simulink model "CylinderSim"  (R2015a)
settings: Solver=ode45  StartTime=0.0  StopTime=2.5  RelTol=1e-3
settings Model: CovSFcnEnable=off  Creator=jportella  LastModifiedBy=user
settings DebuggingCC: SolverPrmCheckMsg=warning

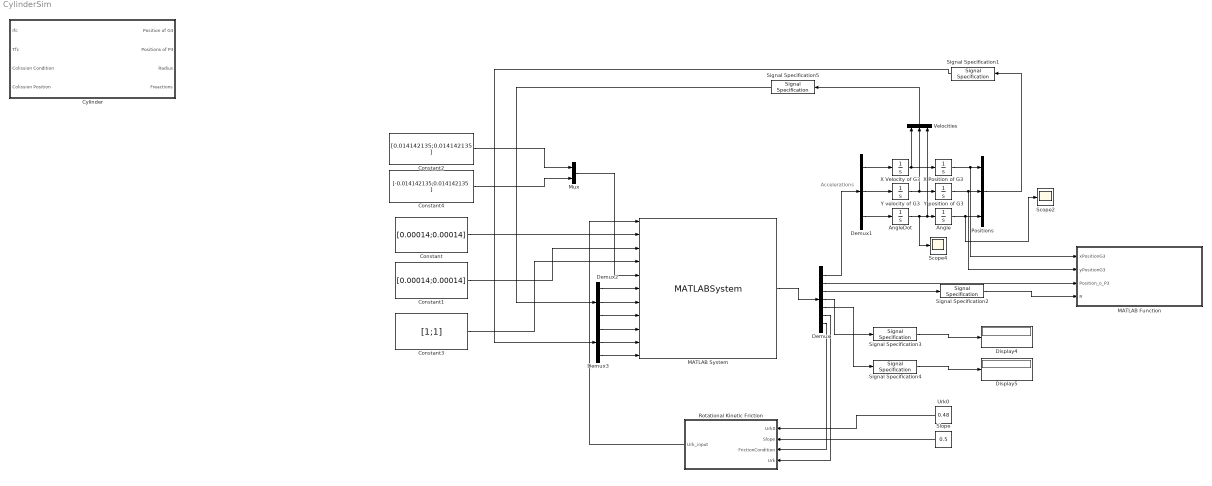
== system CylinderSim ==
  note: Accelerations
  Angle : Integrator
  AngleDot : Integrator
  Constant : Constant  Value=[0.00014;0.00014]
  Constant1 : Constant  Value=[0.00014;0.00014]
  Constant2 : Constant  Value=[0.014142135;0.014142135 ]
  Constant3 : Constant  Value=[1;1]
  Constant4 : Constant  Value=[-0.014142135;0.014142135 ]
  Cylinder : Subsystem
  Demux : Demux  Outputs=7
  Demux1 : Demux  Outputs=3
  Demux2 : Demux  Outputs=3
  Demux3 : Demux  Outputs=3
  Display4 : Display
  Display5 : Display
  MATLAB Function : MATLAB Function  TreatAsAtomicUnit=on
  MATLAB System : MATLABSystem  System=Cylinder  R=0.02  M=0.003  g=9.81  Us=0.5  Uk=0.48  Urs=0.5  Urk=0.48  Ucs=0.5  Uck=0.4  Iz=6.0000000000000008e-07  F_s_x=0.014715  F_s_y=0.014715  F_k_x=0.0141264  F_k_y=0.0141264  T_s=0.0001962  T_k=0.000188352  Position_o_G3=[ 0; 0 ]  Position_G3_P3_frame_cylinder=[0;0.02]  SimulateUsing=Code generation
      mask Type: Cylinder
      mask Display:
      | disp('Cylinder');
      | port_label('input',1,'Urk');
      | port_label('input',2,'IndexFext');
      | port_label('input',3,'ThumbFext');
      | port_label('input',4,'CollisionCondition');
      | port_label('input',5,'CollisionPosition');
      | port_label('input',6,'xDotG3');
      | port_label('input',7,'yDotG3');
      | port_label('input',8,'angleDot');
      | port_label('input',9,'xPositionG3');
      | port_label('input',10,'yPositionG3');
      | port_label('input',11,'angle');
      | port_label('output',1,'CylinderResults');
  Mux : Mux  Inputs=2
  Positions : Mux  Inputs=3
  Rotational Kinetic Friction : Subsystem
  Scope2 : Scope
      settings: SaveName=ScopeData4
  Scope4 : Scope
      settings: SaveName=ScopeData6
  Signal Specification1 : SignalSpecification  Dimensions=3
  Signal Specification2 : SignalSpecification  Dimensions=1
  Signal Specification3 : SignalSpecification  Dimensions=2
  Signal Specification4 : SignalSpecification  Dimensions=2
  Signal Specification5 : SignalSpecification  Dimensions=3
  Slope : Constant  Value=0.5
  Urk0 : Constant  Value=0.48
  Velocities : Mux  Inputs=3
  X Position of G3 : Integrator
  X Velocity of G3 : Integrator
  Y position of G3 : Integrator
  "Y velocity of G3 " : Integrator
  wires:
  X Velocity of G3/1 -> Velocities/1, X Position of G3/1
  AngleDot/1 -> Scope4/1, Velocities/3, Angle/1
  "Y velocity of G3 "/1 -> Velocities/2, Y position of G3/1
  Demux1/1 -> X Velocity of G3/1
  Demux1/2 -> "Y velocity of G3 "/1
  Demux1/3 -> AngleDot/1
  Demux/1 -> Demux1/1
  X Position of G3/1 -> MATLAB Function/1(xPositionG3), Positions/1
  Y position of G3/1 -> MATLAB Function/2(yPositionG3), Positions/2
  Angle/1 -> Scope2/1, Positions/3
  Velocities/1 -> Signal Specification5/1
  Positions/1 -> Signal Specification1/1
  Demux2/1 -> MATLAB System/6
  Demux2/2 -> MATLAB System/7
  Demux2/3 -> MATLAB System/8
  Signal Specification5/1 -> Demux2/1
  Demux3/1 -> MATLAB System/9
  Demux3/2 -> MATLAB System/10
  Demux3/3 -> MATLAB System/11
  Signal Specification1/1 -> Demux3/1
  Demux/3 -> Signal Specification2/1
  Demux/2 -> MATLAB Function/3(Position_o_P3)
  Urk0/1 -> Rotational Kinetic Friction/1(Urk0)
  Slope/1 -> Rotational Kinetic Friction/2(Slope)
  Rotational Kinetic Friction/1(Urk_input) -> MATLAB System/1
  Constant/1 -> MATLAB System/2
  Constant1/1 -> MATLAB System/3
  Constant2/1 -> Mux/1
  Constant4/1 -> Mux/2
  Mux/1 -> MATLAB System/5
  Constant3/1 -> MATLAB System/4
  Demux/6 -> Rotational Kinetic Friction/4(Urk)
  Demux/7 -> Rotational Kinetic Friction/3(FrictionCondition)
  MATLAB System/1 -> Demux/1
  Demux/4 -> Signal Specification3/1
  Signal Specification2/1 -> MATLAB Function/4(R)
  Signal Specification3/1 -> Display4/1
  Signal Specification4/1 -> Display5/1
  Demux/5 -> Signal Specification4/1

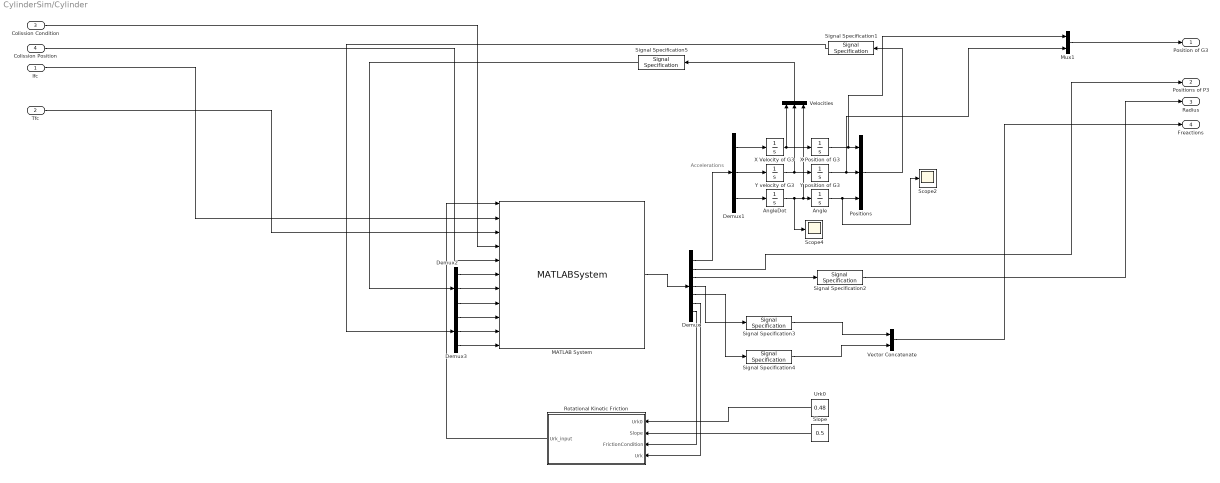
== system CylinderSim/Cylinder ==
  note: Accelerations
  Ifc : Inport
  Tfc : Inport  Port=2
  Colission Condition : Inport  Port=3
  Colission Position : Inport  Port=4
  Angle : Integrator
  AngleDot : Integrator
  Demux : Demux  Outputs=7
  Demux1 : Demux  Outputs=3
  Demux2 : Demux  Outputs=3
  Demux3 : Demux  Outputs=3
  MATLAB System : MATLABSystem  System=Cylinder  R=0.02  M=0.003  g=9.81  Us=0.5  Uk=0.48  Urs=0.5  Urk=0.48  Ucs=0.5  Uck=0.4  Iz=6.0000000000000008e-07  F_s_x=0.014715  F_s_y=0.014715  F_k_x=0.0141264  F_k_y=0.0141264  T_s=0.0001962  T_k=0.000188352  Position_o_G3=[ 0; 0 ]  Position_G3_P3_frame_cylinder=[0;0.02]  SimulateUsing=Code generation
      mask Type: Cylinder
      mask Display:
      | disp('Cylinder');
      | port_label('input',1,'Urk');
      | port_label('input',2,'IndexFext');
      | port_label('input',3,'ThumbFext');
      | port_label('input',4,'CollisionCondition');
      | port_label('input',5,'CollisionPosition');
      | port_label('input',6,'xDotG3');
      | port_label('input',7,'yDotG3');
      | port_label('input',8,'angleDot');
      | port_label('input',9,'xPositionG3');
      | port_label('input',10,'yPositionG3');
      | port_label('input',11,'angle');
      | port_label('output',1,'CylinderResults');
  Mux1 : Mux  Inputs=2
  Positions : Mux  Inputs=3
  Rotational Kinetic Friction : Subsystem
  Scope2 : Scope
  Scope4 : Scope
  Signal Specification1 : SignalSpecification  Dimensions=3
  Signal Specification2 : SignalSpecification  Dimensions=1
  Signal Specification3 : SignalSpecification  Dimensions=2
  Signal Specification4 : SignalSpecification  Dimensions=2
  Signal Specification5 : SignalSpecification  Dimensions=3
  Slope : Constant  Value=0.5
  Urk0 : Constant  Value=0.48
  Vector Concatenate : Concatenate  Mode=Multidimensional array  ConcatenateDimension=2
  Velocities : Mux  Inputs=3
  X Position of G3 : Integrator
  X Velocity of G3 : Integrator
  Y position of G3 : Integrator
  "Y velocity of G3 " : Integrator
  " Position of G3" : Outport
  Positions of P3 : Outport  Port=2
  Radius : Outport  Port=3
  Freactions : Outport  Port=4
  wires:
  X Velocity of G3/1 -> Velocities/1, X Position of G3/1
  AngleDot/1 -> Scope4/1, Velocities/3, Angle/1
  "Y velocity of G3 "/1 -> Velocities/2, Y position of G3/1
  Demux1/1 -> X Velocity of G3/1
  Demux1/2 -> "Y velocity of G3 "/1
  Demux1/3 -> AngleDot/1
  Demux/1 -> Demux1/1
  X Position of G3/1 -> Mux1/1, Positions/1
  Y position of G3/1 -> Mux1/2, Positions/2
  Angle/1 -> Scope2/1, Positions/3
  Velocities/1 -> Signal Specification5/1
  Positions/1 -> Signal Specification1/1
  Demux2/1 -> MATLAB System/6
  Demux2/2 -> MATLAB System/7
  Demux2/3 -> MATLAB System/8
  Signal Specification5/1 -> Demux2/1
  Demux3/1 -> MATLAB System/9
  Demux3/2 -> MATLAB System/10
  Demux3/3 -> MATLAB System/11
  Signal Specification1/1 -> Demux3/1
  Demux/3 -> Signal Specification2/1
  Urk0/1 -> Rotational Kinetic Friction/1(Urk0)
  Slope/1 -> Rotational Kinetic Friction/2(Slope)
  Rotational Kinetic Friction/1(Urk_input) -> MATLAB System/1
  Ifc/1 -> MATLAB System/2
  Tfc/1 -> MATLAB System/3
  Colission Position/1 -> MATLAB System/5
  Colission Condition/1 -> MATLAB System/4
  Demux/6 -> Rotational Kinetic Friction/4(Urk)
  Demux/7 -> Rotational Kinetic Friction/3(FrictionCondition)
  MATLAB System/1 -> Demux/1
  Demux/4 -> Signal Specification3/1
  Signal Specification2/1 -> Radius/1
  Signal Specification3/1 -> Vector Concatenate/1
  Signal Specification4/1 -> Vector Concatenate/2
  Demux/5 -> Signal Specification4/1
  Vector Concatenate/1 -> Freactions/1
  Demux/2 -> Positions of P3/1
  Mux1/1 -> " Position of G3"/1

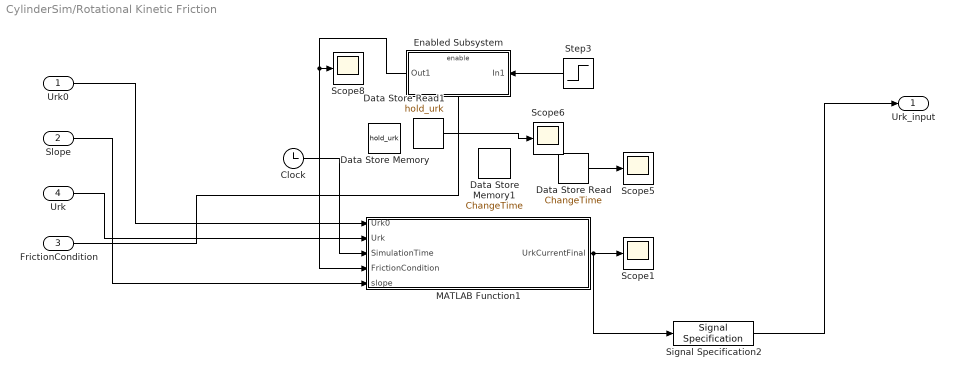
== system CylinderSim/Rotational Kinetic Friction ==
  Urk0 : Inport
  Slope : Inport  Port=2
  FrictionCondition : Inport  Port=3
  Urk : Inport  Port=4
  Clock : Clock
  Data Store Memory : DataStoreMemory  DataStoreName=hold_urk  ReadBeforeWriteMsg=warning  WriteAfterWriteMsg=warning  WriteAfterReadMsg=warning  OutDataTypeStr=double
  Data Store Memory1 : DataStoreMemory  DataStoreName=ChangeTime  ReadBeforeWriteMsg=warning  WriteAfterWriteMsg=warning  WriteAfterReadMsg=warning  OutDataTypeStr=double
  Data Store Read : DataStoreRead  DataStoreName=ChangeTime
  Data Store Read1 : DataStoreRead  DataStoreName=hold_urk
  Enabled Subsystem : Subsystem  TreatAsAtomicUnit=on
  MATLAB Function1 : MATLAB Function  TreatAsAtomicUnit=on
  Scope{1,5..6,8} (4 alike) : Scope
      Scope1 settings: YMax=1  SaveName=ScopeData7
      Scope5 settings: YMax=1  SaveName=ScopeData9
      Scope6 settings: YMax=1  SaveName=ScopeData10
      Scope8 settings: SaveName=ScopeData11
  Signal Specification2 : SignalSpecification  Dimensions=1
  Step3 : Step  Time=0  SampleTime=0
  Urk_input : Outport
  wires:
  MATLAB Function1/1(UrkCurrentFinal) -> Signal Specification2/1, Scope1/1
  Clock/1 -> MATLAB Function1/3(SimulationTime)
  Data Store Read/1 -> Scope5/1
  Data Store Read1/1 -> Scope6/1
  Step3/1 -> Enabled Subsystem/1(In1)
  Enabled Subsystem/1(Out1) -> MATLAB Function1/4(FrictionCondition), Scope8/1
  FrictionCondition/1 -> Enabled Subsystem/Enable
  Urk0/1 -> MATLAB Function1/1(Urk0)
  Urk/1 -> MATLAB Function1/2(Urk)
  Slope/1 -> MATLAB Function1/5(slope)
  Signal Specification2/1 -> Urk_input/1

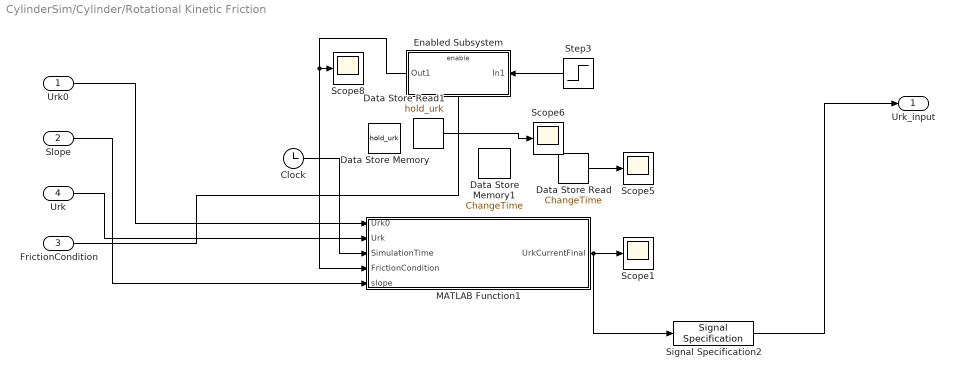
== system CylinderSim/Cylinder/Rotational Kinetic Friction ==
  Urk0 : Inport
  Slope : Inport  Port=2
  FrictionCondition : Inport  Port=3
  Urk : Inport  Port=4
  Clock : Clock
  Data Store Memory : DataStoreMemory  DataStoreName=hold_urk  ReadBeforeWriteMsg=warning  WriteAfterWriteMsg=warning  WriteAfterReadMsg=warning  OutDataTypeStr=double
  Data Store Memory1 : DataStoreMemory  DataStoreName=ChangeTime  ReadBeforeWriteMsg=warning  WriteAfterWriteMsg=warning  WriteAfterReadMsg=warning  OutDataTypeStr=double
  Data Store Read : DataStoreRead  DataStoreName=ChangeTime
  Data Store Read1 : DataStoreRead  DataStoreName=hold_urk
  Enabled Subsystem : Subsystem  TreatAsAtomicUnit=on
  MATLAB Function1 : MATLAB Function  TreatAsAtomicUnit=on
  Scope{1,5..6,8} (4 alike) : Scope
      Scope1 settings: YMax=1  SaveName=ScopeData7
      Scope5 settings: YMax=1  SaveName=ScopeData9
      Scope6 settings: YMax=1  SaveName=ScopeData10
      Scope8 settings: SaveName=ScopeData11
  Signal Specification2 : SignalSpecification  Dimensions=1
  Step3 : Step  Time=0  SampleTime=0
  Urk_input : Outport
  wires:
  MATLAB Function1/1(UrkCurrentFinal) -> Signal Specification2/1, Scope1/1
  Clock/1 -> MATLAB Function1/3(SimulationTime)
  Data Store Read/1 -> Scope5/1
  Data Store Read1/1 -> Scope6/1
  Step3/1 -> Enabled Subsystem/1(In1)
  Enabled Subsystem/1(Out1) -> MATLAB Function1/4(FrictionCondition), Scope8/1
  FrictionCondition/1 -> Enabled Subsystem/Enable
  Urk0/1 -> MATLAB Function1/1(Urk0)
  Urk/1 -> MATLAB Function1/2(Urk)
  Slope/1 -> MATLAB Function1/5(slope)
  Signal Specification2/1 -> Urk_input/1

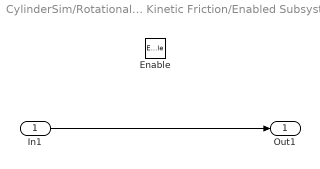
== system CylinderSim/Rotational Kinetic Friction/Enabled Subsystem ==
  In1 : Inport
  Enable : EnablePort
  Out1 : Outport
  wires:
  In1/1 -> Out1/1

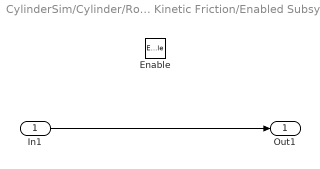
== system CylinderSim/Cylinder/Rotational Kinetic Friction/Enabled Subsystem ==
  In1 : Inport
  Enable : EnablePort
  Out1 : Outport
  wires:
  In1/1 -> Out1/1

== matlab function CylinderSim/MATLAB Function ==
  data: xPositionG3 input; yPositionG3 input; Position_o_P3 input; R input
function DrawCylinder(xPositionG3,yPositionG3,Position_o_P3,R)
%#
    figure(2);
    clf;
    t=linspace(0,2*pi,360);
    plot(xPositionG3,yPositionG3,'r*');
    hold on
    plot(Position_o_P3(1),Position_o_P3(2),'r*');
    x=xPositionG3+R*cos(t);
    y=yPositionG3+R*sin(t);
    plot(x,y,'b');
    hold off
    axis([-0.4 0.4 -0.3 0.3]);
end

== matlab function CylinderSim/Rotational Kinetic Friction/MATLAB Function1 ==
  data: Urk0 input; Urk input; SimulationTime input; UrkCurrentFinal output; FrictionCondition input; slope input; hold_urk data_store_memory; ChangeTime data_store_memory
function UrkCurrentFinal = UrkCurrentCalc(Urk0,Urk,SimulationTime,FrictionCondition,slope)
%#codegen
global hold_urk ChangeTime;
if(SimulationTime==0)
    UrkCurrent=Urk0;
    hold_urk=Urk0;
else
    if(FrictionCondition==1)
        UrkCurrent=(hold_urk-(SimulationTime-ChangeTime)*slope);
    else
        hold_urk=Urk;
        ChangeTime=SimulationTime;
        UrkCurrent=Urk0;
    end
end
if(UrkCurrent>=0)
    UrkCurrentFinal=UrkCurrent;
else
    UrkCurrentFinal=0;
end
end

== matlab function CylinderSim/Cylinder/Rotational Kinetic Friction/MATLAB Function1 ==
  data: Urk0 input; Urk input; SimulationTime input; UrkCurrentFinal output; FrictionCondition input; slope input; hold_urk data_store_memory; ChangeTime data_store_memory
function UrkCurrentFinal = UrkCurrentCalc(Urk0,Urk,SimulationTime,FrictionCondition,slope)
%#codegen
global hold_urk ChangeTime;
if(SimulationTime==0)
    UrkCurrent=Urk0;
    hold_urk=Urk0;
else
    if(FrictionCondition==1)
        UrkCurrent=(hold_urk-(SimulationTime-ChangeTime)*slope);
    else
        hold_urk=Urk;
        ChangeTime=SimulationTime;
        UrkCurrent=Urk0;
    end
end
if(UrkCurrent>=0)
    UrkCurrentFinal=UrkCurrent;
else
    UrkCurrentFinal=0;
end
end
